simulink model "TFlex_SSGP"  (R2018b)
settings: Solver=VariableStepAuto  StartTime=0.0  StopTime=t_end  RelTol=1e-3
values from neighbouring files (symbols this model uses):
  alpha = 1    [TFlex_SSGP_init.m]
  b_init = b    [TFlex_SSGP_init.m]
  beta_init = 0.2    [TFlex_SSGP_init.m]
  beta_min = 0.0000    (= 0)    [TFlex_SSGP_init.m]
  beta_reduc = 0.9    [TFlex_SSGP_init.m]
  bufferResamp = 50    [TFlex_SSGP_init.m]
  bufferSize = 25    [TFlex_SSGP_init.m]
  hyp = abs(hyp_sn(1:end-1))    [TFlex_SSGP_init.m]
  jitter = 1e-4    (= 0.0001)    [TFlex_SSGP_init.m]
  Ma = length(b)    [TFlex_SSGP_init.m]
  ma_init = ma    [TFlex_SSGP_init.m]
  Mb = length(b)    [TFlex_SSGP_init.m]
  mu_X = mean(xTrain')    [TFlex_SSGP_init.m]
  mu_Y = mean(yTrain')    [TFlex_SSGP_init.m]
  Saa_init = Saa    [TFlex_SSGP_init.m]
  sig_X = std(xTrain')    [TFlex_SSGP_init.m]
  sig_Y = std(yTrain')    [TFlex_SSGP_init.m]
  sn = abs(hyp_sn(end))    [TFlex_SSGP_init.m]
  t_hypUpdate = [10 100]    [TFlex_SSGP_init.m]
  t_predict = 20    [TFlex_SSGP_init.m]
  ts = 1/1000    (= 0.001)    [TFlex_SSGP_init.m]
  ts_opti = ts*1000    (= 1)    [TFlex_SSGP_init.m]
  X = xTrain    [TFlex_SSGP_init.m]
  Y = yTrain    [TFlex_SSGP_init.m]
  Z = bufferSize*bufferResamp    (= 1250)    [TFlex_SSGP_init.m]
undefined symbols (not defined in the file or in its folder): Cogging, DiscIntNeverNeededParam, dof, I_limit, PID, Plant, Reference, SVF
libraries: dspmtrx3 x8, simulink x3, dspindex x2
settings Model: Creator=wout7  LastModifiedBy=wout7

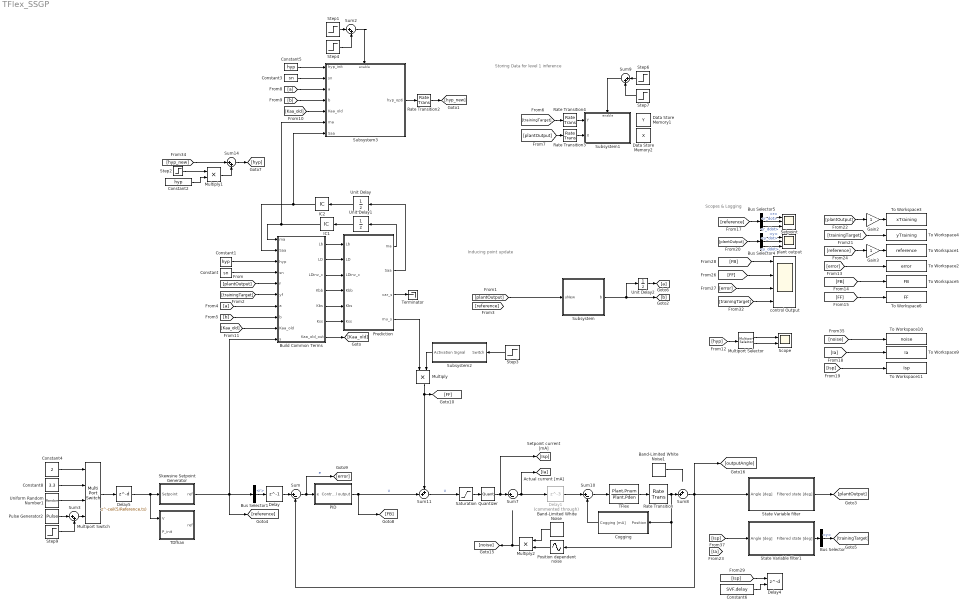
== system TFlex_SSGP ==
  note: Scopes & Logging
  note: Inducing point update
  note: Storing Data for level 1 inference
  Band-Limited White Noise : simulink/Sources/Band-Limited White Noise  Cov=[1e-3]  Ts=ts  seed=48124
  Band-Limited White Noise1 : simulink/Sources/Band-Limited White Noise  Cov=[1e-15]  Ts=ts  seed=[23341]
  Build Common Terms : Subsystem
  Bus Selector : BusSelector  OutputSignals=y
  Bus Selector1 : BusSelector  OutputSignals=r
  Bus Selector4 : BusSelector  OutputSignals=y,y_dot,y_ddot
  Bus Selector5 : BusSelector  OutputSignals=r,r_dot,r_ddot
  Cogging : Subsystem
  Constant : Constant  Value=sn
  Constant1 : Constant  Value=hyp
  Constant2 : Constant  Value=hyp  SampleTime=ts_opti
  Constant3 : Constant  Value=sn  SampleTime=ts_opti
  Constant4 : Constant  Value=2  SampleTime=Reference.ts
  Constant5 : Constant  Value=hyp
  Constant6 : Constant  Value=SVF.delay  SampleTime=ts
  Constant8 : Constant  Value=3.3  SampleTime=Reference.ts
  Data Store Memory1 : DataStoreMemory  DataStoreName=Y  ReadBeforeWriteMsg=warning  WriteAfterWriteMsg=warning  WriteAfterReadMsg=warning  InitialValue=zeros(bufferSize,1)  VectorParams1D=off  ShowAdditionalParam=off  OutDataTypeStr=double
      settings: LockScale=on
  Data Store Memory2 : DataStoreMemory  DataStoreName=X  ReadBeforeWriteMsg=warning  WriteAfterWriteMsg=warning  WriteAfterReadMsg=warning  InitialValue=zeros(bufferSize,3)  VectorParams1D=off  ShowAdditionalParam=off  OutDataTypeStr=double
      settings: LockScale=on
  Delay : Delay  DelayLength=1
  Delay1 : Delay  Commented=through  DelayLength=3  InitialCondition=0
  Delay4 : Delay  DelayLengthSource=Input port  DelayLength=3  InitialCondition=0
      settings: InputPortMap=u0,p1
  Delay5 : Delay  DelayLength=ceil(5/Reference.ts)  SampleTime=Reference.ts
  Gain2 : Gain
  Gain3 : Gain
  IC1 : InitialCondition  Value=ma_init
  IC2 : InitialCondition  Value=Saa_init
  Multiply : Product
  Multiply1 : Product
  Multiply2 : Product
  Multiport Selector : dspindex/Multiport Selector  rowsOrCols=Columns  idxCellArray={ 1:3,4}  idxErrMode=Clip Index
  Multiport Switch : MultiPortSwitch
  PID : Subsystem
  Position dependent noise : Sin  TimeSource=Use external signal  Amplitude=2.5  Bias=7.4979  Frequency=2*pi/13  SampleTime=0
  Prediction : Subsystem
  Pulse Generator2 : DiscretePulseGenerator  Amplitude=2*24  SampleTime=Reference.ts
  Quantizer : Quantizer  QuantizationInterval=1
  Rate Transition : RateTransition  OutPortSampleTime=ts
  Rate Transition2 : RateTransition  OutPortSampleTime=ts
  Rate Transition3 : RateTransition  OutPortSampleTime=ts*bufferResamp
  Rate Transition4 : RateTransition  OutPortSampleTime=ts*bufferResamp
  Saturation : Saturate  UpperLimit=I_limit  LowerLimit=-I_limit
  Scope : Scope  NumInputPorts=2
  Setpoint : Scope  NumInputPorts=3
  Skewsine Setpoint Generator : Subsystem
  State Variable filter : Subsystem
  State Variable filter1 : Subsystem
  Step1 : Step  Time=t_hypUpdate(2)  After=-1  SampleTime=ts_opti
  Step2 : Step  Time=t_hypUpdate(1)+ts  Before=1  After=0  SampleTime=ts_opti
  Step3 : Step  Time=t_predict  SampleTime=0
  Step4 : Step  Time=t_hypUpdate(1)  SampleTime=ts_opti
  Step6 : Step  Time=t_hypUpdate(2)  After=-1  SampleTime=ts_opti
  Step7 : Step  Time=t_hypUpdate(1)-Z*ts  SampleTime=ts_opti
  Step9 : Step  Time=0  After=-24  SampleTime=Reference.ts
  Subsystem : Subsystem
  Subsystem1 : Subsystem
  Subsystem2 : Subsystem
  Subsystem3 : Subsystem
  Sum : Sum  Inputs=|+-
  Sum10 : Sum  Inputs=|+-
  Sum11 : Sum  Inputs=++|
  Sum{2..3,9,14} (4 alike) : Sum  Inputs=|++
  Sum7 : Sum  Inputs=|+-
  Sum8 : Sum  Inputs=++|
  TDfhan : Subsystem
  TFlex : TransferFcn  Numerator=Plant.Pnum  Denominator=Plant.Pden  ContinuousStateAttributes='angle'
  Terminator : Terminator
  To Workspace1 : ToWorkspace  VariableName=reference  SampleTime=-1
  To Workspace10 : ToWorkspace  VariableName=noise  SampleTime=-1
  To Workspace11 : ToWorkspace  VariableName=Isp  SampleTime=-1
  To Workspace2 : ToWorkspace  VariableName=error  SampleTime=-1
  To Workspace3 : ToWorkspace  VariableName=xTraining  SampleTime=-1
  To Workspace4 : ToWorkspace  VariableName=yTraining  SampleTime=-1
  To Workspace5 : ToWorkspace  VariableName=FB  SampleTime=-1
  To Workspace6 : ToWorkspace  VariableName=FF  SampleTime=-1
  To Workspace9 : ToWorkspace  VariableName=Ia  SampleTime=-1
  Uniform Random Number1 : UniformRandomNumber  Minimum=-23  Maximum=23  Seed=Reference.seed  SampleTime=Reference.ts
  Unit Delay : UnitDelay  SampleTime=-1
  Unit Delay1 : UnitDelay  SampleTime=-1
  Unit Delay2 : UnitDelay  SampleTime=-1
  control Output : Scope  NumInputPorts=4
  plant output : Scope  NumInputPorts=3
  wires:
  Sum/1 -> [error], PID/1(e)  "e"
  Sum8/1 -> [outputAngle], Sum/2, State Variable filter/1(Angle [deg])
  Bus Selector1/1 -> Delay/1  "<r>"
  TFlex/1 -> Rate Transition/1
  [reference] -> Gain3/1
  Bus Selector5/2 -> Setpoint/2  "<r_dot>"
  Bus Selector5/1 -> Setpoint/1  "<r>"
  [error] -> To Workspace2/1
  Bus Selector5/3 -> Setpoint/3  "<r_ddot>"
  [FB] -> To Workspace5/1
  [plantOutput] -> Gain2/1
  Gain2/1 -> To Workspace3/1
  [plantOutput] -> Bus Selector4/1
  Gain3/1 -> To Workspace1/1
  Bus Selector4/1 -> plant output/1  "<y>"
  Bus Selector4/3 -> plant output/3  "<y_ddot>"
  [reference] -> Bus Selector5/1
  [trainingTarget] -> To Workspace4/1
  Bus Selector4/2 -> plant output/2  "<y_dot>"
  [FF] -> To Workspace6/1
  [trainingTarget] -> control Output/4
  [FF] -> control Output/2
  [error] -> control Output/3
  [FB] -> control Output/1
  Saturation/1 -> Quantizer/1
  PID/1(Control output) -> Sum11/2, [FB]  "u"
  State Variable filter/1(Filtered state [deg]) -> [plantOutput]
  Rate Transition/1 -> Sum8/2, Cogging/1(Position), Position dependent noise/1
  Constant6/1 -> Delay4/2
  Sum11/1 -> Saturation/1  "u"
  [Isp] -> Delay4/1
  Sum10/1 -> TFlex/1
  State Variable filter1/1(Filtered state [deg]) -> Bus Selector/1
  Sum7/1 -> Delay1/1, [Ia]
  Multiply2/1 -> [noise]
  Cogging/1(Cogging [mA]) -> Sum10/2
  Quantizer/1 -> [Isp], Sum7/1
  Multiply/1 -> Sum11/1, [FF]
  Band-Limited White Noise/1 -> Multiply2/1
  Position dependent noise/1 -> Multiply2/2
  [noise] -> To Workspace10/1
  [Ia] -> To Workspace9/1
  [Isp] -> To Workspace11/1
  Band-Limited White Noise1/1 -> ?
  Delay1/1 -> Sum10/1
  [Isp] -> State Variable filter1/1(Angle [deg])
  Prediction/1(ma) -> Unit Delay1/1
  Prediction/2(Saa) -> Unit Delay/1
  Unit Delay/1 -> IC2/1
  Unit Delay1/1 -> IC1/1
  Prediction/3(var_s) -> Terminator/1
  [plantOutput] -> Build Common Terms/5(f)
  [trainingTarget] -> Build Common Terms/6(yf)
  Constant/1 -> Build Common Terms/4(sn)
  Constant1/1 -> Build Common Terms/3(hyp)
  [a] -> Build Common Terms/7(a)
  [b] -> Build Common Terms/8(b)
  Build Common Terms/1(Lb) -> Prediction/1(Lb)
  Build Common Terms/2(LD) -> Prediction/2(LD)
  Build Common Terms/3(LDinv_c) -> Prediction/3(LDinv_c)
  Build Common Terms/4("Kbb ") -> Prediction/4(Kbb)
  Build Common Terms/5(Kbs) -> Prediction/5(Kbs)
  Build Common Terms/6(Kss) -> Prediction/6(Kss)
  Bus Selector/1 -> [trainingTarget]  "<y>"
  Unit Delay2/1 -> [a]
  IC1/1 -> Subsystem3/6(ma), Build Common Terms/1(ma)
  Prediction/4(mu_s) -> Multiply/1
  Subsystem2/1(Activation Signal) -> Multiply/2
  Step3/1 -> Subsystem2/1(Switch)
  Subsystem/1(b) -> Unit Delay2/1, [b]
  Constant8/1 -> Multiport Switch/2
  Pulse Generator2/1 -> Sum3/1
  Uniform Random Number1/1 -> Multiport Switch/3
  Sum3/1 -> Multiport Switch/4
  Multiport Switch/1 -> Delay5/1
  Step9/1 -> Sum3/2
  Constant4/1 -> Multiport Switch/1
  Delay5/1 -> Skewsine Setpoint Generator/1(Setpoint), TDfhan/1(V)
  Step7/1 -> Sum9/2
  Sum9/1 -> Subsystem1/Enable
  Rate Transition3/1 -> Subsystem1/2(X)
  Step6/1 -> Sum9/1
  [trainingTarget] -> Rate Transition4/1
  [plantOutput] -> Rate Transition3/1
  Rate Transition4/1 -> Subsystem1/1(Y)
  [a] -> Subsystem3/3(a)
  [b] -> Subsystem3/4(b)
  Build Common Terms/7(Kaa_old_out) -> [Kaa_old]
  [Kaa_old] -> Subsystem3/5(Kaa_old)
  [Kaa_old] -> Build Common Terms/9(Kaa_old)
  Subsystem3/1(hyp_opti) -> Rate Transition2/1
  Constant2/1 -> Multiply1/2
  Sum14/1 -> [hyp]
  Multiply1/1 -> Sum14/2
  [hyp_new] -> Sum14/1
  Step2/1 -> Multiply1/1
  Constant5/1 -> Subsystem3/1(hyp_init)
  Constant3/1 -> Subsystem3/2(sn)
  IC2/1 -> Subsystem3/7(Saa), Build Common Terms/2(Saa)
  Sum2/1 -> Subsystem3/Enable
  Step4/1 -> Sum2/2
  Step1/1 -> Sum2/1
  Rate Transition2/1 -> [hyp_new]
  [hyp] -> Multiport Selector/1
  Multiport Selector/1 -> Scope/1
  Multiport Selector/2 -> Scope/2
  [plantOutput] -> Subsystem/1(uNew)
  Delay/1 -> Sum/1
  Skewsine Setpoint Generator/1(ref) -> Bus Selector1/1, Build Common Terms/10(s), [reference]

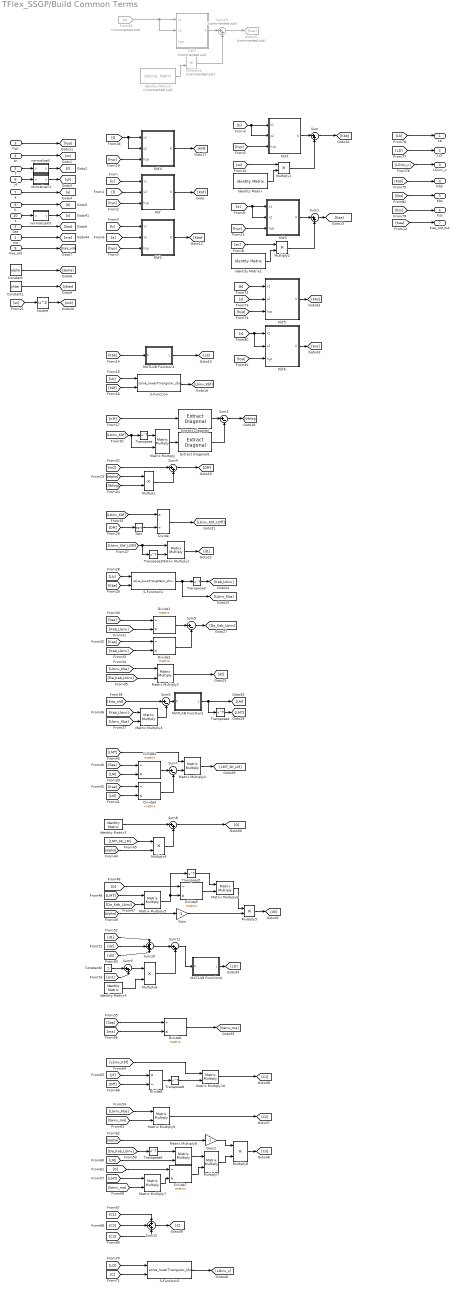
== system TFlex_SSGP/Build Common Terms ==
  ma : Inport  PortDimensions=[Ma,1]
  Saa : Inport  Port=2
  hyp : Inport  Port=3
  sn : Inport  Port=4
  f : Inport  Port=5  PortDimensions=[1,dof]
  yf : Inport  Port=6  PortDimensions=[1,1]
  a : Inport  Port=7
  b : Inport  Port=8
  Kaa_old : Inport  Port=9
  s : Inport  Port=10  PortDimensions=[1,dof]
  Constant : Constant  Value=alpha
  Constant1 : Constant  Value=jitter
  Constant2 : Constant
  Divide : Product  Inputs=*/
  Divide{1..7} (7 alike) : Product  Inputs=/*  Multiplication=Matrix(*)
  Divide8 : Product  Inputs=*/
  Extract Diagonal : dspmtrx3/Extract Diagonal
      settings: SourceProductName=DSP System Toolbox  SourceProductBaseCode=DS
  Extract Diagonal1 : dspmtrx3/Extract Diagonal
      settings: SourceProductName=DSP System Toolbox  SourceProductBaseCode=DS
  From83 : From  Commented=on  GotoTag=a
  Gain : Gain  Gain=-1
  Gain1 : Gain  Gain=-1
  Goto45 : Goto  Commented=on  GotoTag=Kaa
  Identity Matrix : dspmtrx3/Identity Matrix  Inherit=off  N=Mb  Ts=1  dataType=double  isSigned=on  wordLen=16  udDataType=sfix(16)  fracBitsMode=Best precision  numFracBits=15  OutDataTypeStr=double  LastOutDataTypeStr=double
      settings: SourceProductName=DSP System Toolbox
  Identity Matrix1 : dspmtrx3/Identity Matrix  Inherit=off  N=Ma  Ts=1  dataType=double  isSigned=on  wordLen=16  udDataType=sfix(16)  fracBitsMode=Best precision  numFracBits=15  OutDataTypeStr=double  LastOutDataTypeStr=double
      settings: SourceProductName=DSP System Toolbox
  Identity Matrix3 : dspmtrx3/Identity Matrix  Inherit=off  N=Ma  Ts=1  dataType=double  isSigned=on  wordLen=16  udDataType=sfix(16)  fracBitsMode=Best precision  numFracBits=15  OutDataTypeStr=double  LastOutDataTypeStr=double
      settings: SourceProductName=DSP System Toolbox
  Identity Matrix4 : dspmtrx3/Identity Matrix  Inherit=off  N=Mb  Ts=1  dataType=double  isSigned=on  wordLen=16  udDataType=sfix(16)  fracBitsMode=Best precision  numFracBits=15  OutDataTypeStr=double  LastOutDataTypeStr=double
      settings: SourceProductName=DSP System Toolbox
  Identity Matrix5 : dspmtrx3/Identity Matrix  Commented=on  Inherit=off  N=Mb  Ts=1  dataType=double  isSigned=on  wordLen=16  udDataType=sfix(16)  fracBitsMode=Best precision  numFracBits=15  OutDataTypeStr=double  LastOutDataTypeStr=double
      settings: SourceProductName=DSP System Toolbox
  Kbf : MATLAB Function  TreatAsAtomicUnit=on
  Kbf1 : MATLAB Function  TreatAsAtomicUnit=on
  Kbf2 : MATLAB Function  TreatAsAtomicUnit=on
  Kbf3 : MATLAB Function  TreatAsAtomicUnit=on
  Kbf4 : MATLAB Function  TreatAsAtomicUnit=on
  Kbf5 : MATLAB Function  TreatAsAtomicUnit=on
  Kbf6 : MATLAB Function  TreatAsAtomicUnit=on
  Kbf7 : MATLAB Function  Commented=on  TreatAsAtomicUnit=on
  MATLAB Function1 : MATLAB Function  TreatAsAtomicUnit=on
  MATLAB Function2 : MATLAB Function  TreatAsAtomicUnit=on
  MATLAB Function4 : MATLAB Function  TreatAsAtomicUnit=on
  Matrix Multiply{,1..10} (11 alike) : Product  Multiplication=Matrix(*)
  Multiply{,1..2,4..6,8} (7 alike) : Product
  Multiply7 : Product  Multiplication=Matrix(*)
  Multiply9 : Product  Commented=on
  S-Function : S-Function  FunctionName=solve_lowerTriangular_sfun  Parameters=Mb  SFunctionDeploymentMode=off  EnableBusSupport=off
  S-Function1 : S-Function  FunctionName=solve_lowerTriangMatrix_sfun  Parameters=Mb  SFunctionDeploymentMode=off  EnableBusSupport=off
  S-Function2 : S-Function  FunctionName=solve_lowerTriangular_sfun  Parameters=Mb  SFunctionDeploymentMode=off  EnableBusSupport=off
  Sqrt : Sqrt  SaturateOnIntegerOverflow=on
  Square : Math  Operator=square  SaturateOnIntegerOverflow=on
  Sum{,1,4,8..9,11} (6 alike) : Sum  Inputs=|++
  Sum10 : Sum  Inputs=+++
  Sum12 : Sum  Inputs=+++
  Sum13 : Sum  Commented=on  Inputs=|++
  Sum{3,5..7} (4 alike) : Sum  Inputs=|+-
  Transpose{,2..6,8} (7 alike) : Math  Operator=transpose  SaturateOnIntegerOverflow=on
  normalizeX : MATLAB Function  TreatAsAtomicUnit=on
  normalizeX3 : MATLAB Function  TreatAsAtomicUnit=on
  normalizeY1 : MATLAB Function  TreatAsAtomicUnit=on
  Lb : Outport
  LD : Outport  Port=2
  LDinv_c : Outport  Port=3
  "Kbb " : Outport  Port=4
  Kbs : Outport  Port=5
  Kss : Outport  Port=6
  Kaa_old_out : Outport  Port=7
  wires:
  Saa/1 -> [Saa]
  yf/1 -> normalizeY1/1(u)
  f/1 -> normalizeX/1(u)
  sn/1 -> [sn]
  hyp/1 -> [hyp]
  Constant/1 -> [alpha]
  Constant1/1 -> [jitter]
  [b] -> Kbf/1(x1)
  [f] -> Kbf/2(x2)
  [hyp] -> Kbf/3(hyp)
  Kbf/1(K) -> [Kbf]
  [hyp] -> Kbf1/3(hyp)
  [b] -> Kbf1/2(x2), Kbf1/1(x1)
  Multiply1/1 -> Sum/2
  Identity Matrix/1 -> Multiply1/2
  [sn] -> Multiply1/1
  Kbf1/1(K) -> Sum/1
  Sum/1 -> [Kbb]
  [hyp] -> Kbf2/3(hyp)
  [a] -> Kbf2/2(x2)
  [b] -> Kbf2/1(x1)
  Kbf2/1(K) -> [Kba]
  [hyp] -> Kbf3/3(hyp)
  [a] -> Kbf3/2(x2), Kbf3/1(x1)
  Multiply2/1 -> Sum1/2
  [sn] -> Multiply2/1
  Identity Matrix1/1 -> Multiply2/2
  Kbf3/1(K) -> Sum1/1
  Sum1/1 -> [Kaa]
  [Kbb] -> MATLAB Function1/1(K)
  MATLAB Function1/1(L) -> [Lb]
  [Lb] -> S-Function/1
  [Kbf] -> S-Function/2
  S-Function/1 -> [Lbinv_Kbf]
  [hyp] -> Kbf4/3(hyp)
  Kbf4/1(K) -> [Kff]
  [f] -> Kbf4/2(x2), Kbf4/1(x1)
  [Kff] -> Extract Diagonal/1
  [Lbinv_Kbf] -> Matrix Multiply/2, Transpose/1
  Transpose/1 -> Matrix Multiply/1
  Matrix Multiply/1 -> Extract Diagonal1/1
  Extract Diagonal/1 -> Sum3/1
  Sum3/1 -> [Qfdiag]
  Extract Diagonal1/1 -> Sum3/2
  [sn] -> Square/1
  Square/1 -> [sn2]
  [alpha] -> Multiply/1
  [Qfdiag] -> Multiply/2
  Multiply/1 -> Sum4/2
  [sn2] -> Sum4/1
  Sum4/1 -> [Dff]
  [Lbinv_Kbf] -> Divide/1
  Sqrt/1 -> Divide/2
  Divide/1 -> [Lbinv_Kbf_LDff]
  Transpose2/1 -> Matrix Multiply1/2
  [Lbinv_Kbf_LDff] -> Transpose2/1, Matrix Multiply1/1
  Matrix Multiply1/1 -> [d1]
  [Lb] -> S-Function1/1
  [Kba] -> S-Function1/2
  Transpose3/1 -> [Kab_Lbinv]
  S-Function1/1 -> Transpose3/1, [Lbinv_Kba]
  [Saa] -> Divide1/1
  [Kab_Lbinv] -> Divide1/2
  Divide1/1 -> Sum5/1
  Divide2/1 -> Sum5/2
  [Kab_Lbinv] -> Divide2/2
  [Kaa] -> Divide2/1
  Sum5/1 -> [Da_Kab_Lbinv]
  [Da_Kab_Lbinv] -> Matrix Multiply2/2
  [Lbinv_Kba] -> Matrix Multiply2/1
  Matrix Multiply2/1 -> [d2]
  [Lbinv_Kba] -> Matrix Multiply3/2
  [Kab_Lbinv] -> Matrix Multiply3/1
  Matrix Multiply3/1 -> Sum6/2
  [Kaa_old] -> Sum6/1
  Sum6/1 -> MATLAB Function2/1(K)
  MATLAB Function2/1(L) -> [LM], Transpose4/1
  Transpose4/1 -> [LMT]
  [LM] -> Divide3/2
  [Saa] -> Divide3/1
  [Kaa] -> Divide4/1
  [LM] -> Divide4/2
  Divide3/1 -> Sum7/1
  Divide4/1 -> Sum7/2
  Sum7/1 -> Matrix Multiply4/2
  Matrix Multiply4/1 -> [LMT_SK_LM]
  [LMT] -> Matrix Multiply4/1
  Identity Matrix3/1 -> Sum8/1
  [alpha] -> Multiply4/2
  [LMT_SK_LM] -> Multiply4/1
  Multiply4/1 -> Sum8/2
  Sum8/1 -> [Q]
  [LMT] -> Matrix Multiply5/1
  [Da_Kab_Lbinv] -> Matrix Multiply5/2
  Matrix Multiply5/1 -> Transpose5/1, Divide5/2
  [Q] -> Divide5/1
  Divide5/1 -> Matrix Multiply6/2
  Transpose5/1 -> Matrix Multiply6/1
  Matrix Multiply6/1 -> Multiply5/1
  [alpha] -> Gain/1
  Gain/1 -> Multiply5/2
  Multiply5/1 -> [d3]
  Constant2/1 -> Sum9/1
  [sn2] -> Sum9/2
  Sum9/1 -> Multiply6/1
  Identity Matrix4/1 -> Multiply6/2
  [d2] -> Sum10/2
  [d3] -> Sum10/3
  [d1] -> Sum10/1
  Sum10/1 -> Sum11/1
  Multiply6/1 -> Sum11/2
  Sum11/1 -> MATLAB Function4/1(K)
  MATLAB Function4/1(L) -> [LD]
  [Saa] -> Divide6/1
  [ma] -> Divide6/2
  Divide6/1 -> [Sainv_ma]
  [LMT] -> Matrix Multiply7/1
  [Sainv_ma] -> Matrix Multiply7/2
  [Da_Kab_Lbinv] -> Transpose6/1
  Transpose6/1 -> Matrix Multiply8/1
  [LM] -> Matrix Multiply8/2
  [Q] -> Divide7/1
  Matrix Multiply7/1 -> Divide7/2
  Matrix Multiply8/1 -> Multiply7/1
  Divide7/1 -> Multiply7/2
  Multiply7/1 -> Multiply8/2
  [alpha] -> Gain1/1
  Gain1/1 -> Multiply8/1
  Multiply8/1 -> [C3]
  [Lbinv_Kba] -> Matrix Multiply9/1
  [Sainv_ma] -> Matrix Multiply9/2
  Matrix Multiply9/1 -> [C2]
  [yf] -> Divide8/1
  [Dff] -> Divide8/2
  Divide8/1 -> Transpose8/1
  [Lbinv_Kbf] -> Matrix Multiply10/1
  Transpose8/1 -> Matrix Multiply10/2
  Matrix Multiply10/1 -> [C1]
  [C2] -> Sum12/2
  [C1] -> Sum12/1
  [C3] -> Sum12/3
  Sum12/1 -> [C]
  [LD] -> S-Function2/1
  [C] -> S-Function2/2
  S-Function2/1 -> [LDinv_c]
  s/1 -> normalizeX3/1(u)
  [b] -> Kbf5/1(x1)
  [s] -> Kbf5/2(x2)
  [hyp] -> Kbf5/3(hyp)
  Kbf5/1(K) -> [Kbs]
  [Kbb] -> "Kbb "/1
  [LDinv_c] -> LDinv_c/1
  [LD] -> LD/1
  [Lb] -> Lb/1
  [Kbs] -> Kbs/1
  a/1 -> [a]
  b/1 -> [b]
  normalizeX3/1(y) -> [s]
  ma/1 -> [ma]
  normalizeY1/1(y) -> [yf]
  [Dff] -> Sqrt/1
  Kbf6/1(K) -> [Kss]
  [hyp] -> Kbf6/3(hyp)
  [s] -> Kbf6/1(x1), Kbf6/2(x2)
  [Kss] -> Kss/1
  ? -> Kbf7/3(hyp)
  Identity Matrix5/1 -> Multiply9/2
  From83/1 -> Kbf7/2(x2), Kbf7/1(x1)
  Multiply9/1 -> Sum13/2
  ? -> Multiply9/1
  Kbf7/1(K) -> Sum13/1
  Sum13/1 -> Goto45/1
  normalizeX/1(y) -> [f]
  Kaa_old/1 -> [Kaa_old]
  [Kaa] -> Kaa_old_out/1

== system TFlex_SSGP/Cogging ==
  Position : Inport
  Gain : Gain  Gain=20
  Scope : Scope
  Sine Wave Function : Sin  TimeSource=Use external signal  Amplitude=Cogging.amplitude  Frequency=2*pi./Cogging.frequency  Phase=Cogging.phase*2*pi  SampleTime=0
  Sum of Elements : Sum  Inputs=+
  Cogging [mA] : Outport
  wires:
  Gain/1 -> Scope/1, [Cogging], Cogging [mA]/1
  Sum of Elements/1 -> Gain/1
  Position/1 -> Sine Wave Function/1
  Sine Wave Function/1 -> Sum of Elements/1

== system TFlex_SSGP/PID ==
  e : Inport
  Discrete Derivative : simulink/Discrete/Discrete Derivative  gainval=1.0  ICPrevScaledInput=0.0  OutMin=[]  OutMax=[]  OutDataType=fixdt(1, 16)  OutScaling=2^-10  DoSatur=off
  Discrete-Time Integrator2 : DiscreteIntegrator  SampleTime=-1  ICPrevOutput=DiscIntNeverNeededParam  ICPrevScaledInput=DiscIntNeverNeededParam
  Gain1 : Gain  Gain=PID.Kp
  Gain2 : Gain  Gain=PID.Ki
  Gain3 : Gain  Gain=PID.Kd
  Lowpass : DiscreteTransferFcn  Numerator=PID.LPnum  Denominator=PID.LPden  SampleTime=ts
  Sum2 : Sum  Inputs=3
  Control output : Outport
  wires:
  Discrete-Time Integrator2/1 -> Gain2/1
  Gain1/1 -> Sum2/2
  Gain2/1 -> Sum2/1
  Gain3/1 -> Sum2/3
  Sum2/1 -> Control output/1
  e/1 -> Discrete-Time Integrator2/1, Gain1/1, Lowpass/1
  Lowpass/1 -> Discrete Derivative/1
  Discrete Derivative/1 -> Gain3/1

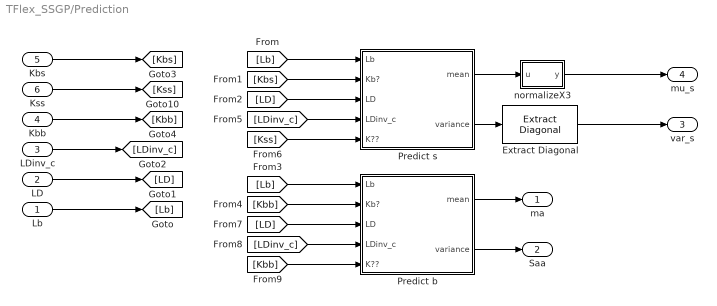
== system TFlex_SSGP/Prediction ==
  Lb : Inport
  LD : Inport  Port=2
  LDinv_c : Inport  Port=3
  Kbb : Inport  Port=4
  Kbs : Inport  Port=5
  Kss : Inport  Port=6
  Extract Diagonal : dspmtrx3/Extract Diagonal
      settings: SourceProductName=DSP System Toolbox  SourceProductBaseCode=DS
  Predict b : Subsystem
  Predict s : Subsystem
  normalizeX3 : MATLAB Function  TreatAsAtomicUnit=on
  ma : Outport
  Saa : Outport  Port=2
  var_s : Outport  Port=3
  mu_s : Outport  Port=4
  wires:
  Kbs/1 -> [Kbs]
  Kss/1 -> [Kss]
  Extract Diagonal/1 -> var_s/1
  [Lb] -> Predict s/1(Lb)
  [Kbs] -> Predict s/2(Kb?)
  [LD] -> Predict s/3(LD)
  [LDinv_c] -> Predict s/4(LDinv_c)
  [Kss] -> Predict s/5(K??)
  Predict s/1(mean) -> normalizeX3/1(u)
  Predict s/2(variance) -> Extract Diagonal/1
  [Kbb] -> Predict b/2(Kb?)
  [Kbb] -> Predict b/5(K??)
  [LDinv_c] -> Predict b/4(LDinv_c)
  [LD] -> Predict b/3(LD)
  Predict b/2(variance) -> Saa/1
  [Lb] -> Predict b/1(Lb)
  Predict b/1(mean) -> ma/1
  Lb/1 -> [Lb]
  Kbb/1 -> [Kbb]
  LDinv_c/1 -> [LDinv_c]
  LD/1 -> [LD]
  normalizeX3/1(y) -> mu_s/1

== system TFlex_SSGP/Skewsine Setpoint Generator ==
  Setpoint : Inport
  Bus Creator : BusCreator  Inputs=3
  Subsystem : Subsystem
  ref : Outport
  wires:
  Subsystem/3(r_ddot) -> Bus Creator/3  "r_ddot"
  Bus Creator/1 -> ref/1
  Subsystem/2(r_dot) -> Bus Creator/2  "r_dot"
  Subsystem/1(r) -> Bus Creator/1  "r"
  Setpoint/1 -> Subsystem/1(setpoint)

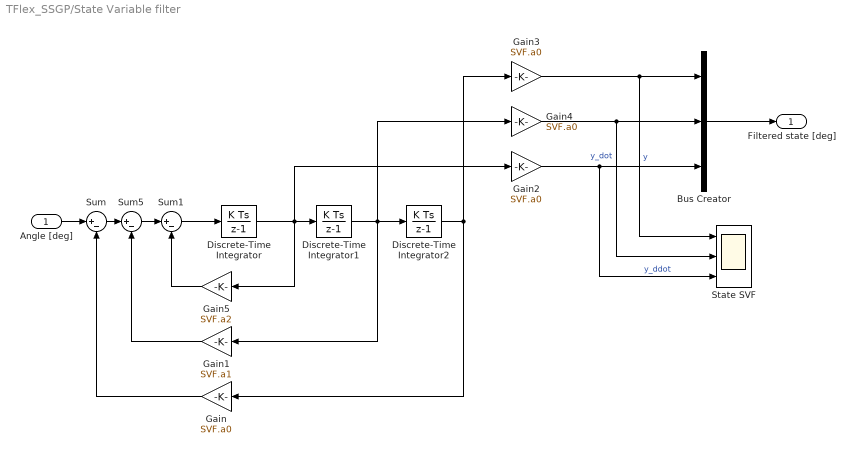
== system TFlex_SSGP/State Variable filter ==
  Angle [deg] : Inport
  Bus Creator : BusCreator  Inputs=3
  Discrete-Time Integrator : DiscreteIntegrator  SampleTime=-1  ICPrevOutput=DiscIntNeverNeededParam  ICPrevScaledInput=DiscIntNeverNeededParam
  Discrete-Time Integrator1 : DiscreteIntegrator  SampleTime=-1  ICPrevOutput=DiscIntNeverNeededParam  ICPrevScaledInput=DiscIntNeverNeededParam
  Discrete-Time Integrator2 : DiscreteIntegrator  SampleTime=-1  ICPrevOutput=DiscIntNeverNeededParam  ICPrevScaledInput=DiscIntNeverNeededParam
  Gain{,2..4} (4 alike) : Gain  Gain=SVF.a0
  Gain1 : Gain  Gain=SVF.a1
  Gain5 : Gain  Gain=SVF.a2
  State SVF : Scope  NumInputPorts=3
  Sum : Sum  Inputs=|+-
  Sum1 : Sum  Inputs=|+-
  Sum5 : Sum  Inputs=|+-
  Filtered state [deg] : Outport  SampleTime=ts
  wires:
  Bus Creator/1 -> Filtered state [deg]/1
  Sum1/1 -> Discrete-Time Integrator/1
  Angle [deg]/1 -> Sum/1
  Sum/1 -> Sum5/1
  Gain/1 -> Sum/2
  Gain1/1 -> Sum5/2
  Gain3/1 -> State SVF/1, Bus Creator/1  "y"
  Gain2/1 -> State SVF/3, Bus Creator/3  "y_ddot"
  Gain4/1 -> State SVF/2, Bus Creator/2  "y_dot"
  Gain5/1 -> Sum1/2
  Sum5/1 -> Sum1/1
  Discrete-Time Integrator/1 -> Discrete-Time Integrator1/1, Gain2/1, Gain5/1
  Discrete-Time Integrator1/1 -> Discrete-Time Integrator2/1, Gain4/1, Gain1/1
  Discrete-Time Integrator2/1 -> Gain3/1, Gain/1

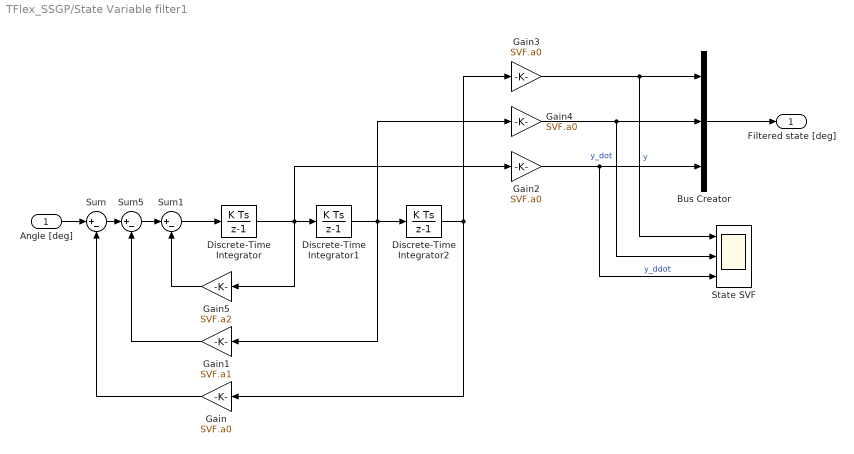
== system TFlex_SSGP/State Variable filter1 ==
  Angle [deg] : Inport
  Bus Creator : BusCreator  Inputs=3
  Discrete-Time Integrator : DiscreteIntegrator  SampleTime=-1  ICPrevOutput=DiscIntNeverNeededParam  ICPrevScaledInput=DiscIntNeverNeededParam
  Discrete-Time Integrator1 : DiscreteIntegrator  SampleTime=-1  ICPrevOutput=DiscIntNeverNeededParam  ICPrevScaledInput=DiscIntNeverNeededParam
  Discrete-Time Integrator2 : DiscreteIntegrator  SampleTime=-1  ICPrevOutput=DiscIntNeverNeededParam  ICPrevScaledInput=DiscIntNeverNeededParam
  Gain{,2..4} (4 alike) : Gain  Gain=SVF.a0
  Gain1 : Gain  Gain=SVF.a1
  Gain5 : Gain  Gain=SVF.a2
  State SVF : Scope  NumInputPorts=3
  Sum : Sum  Inputs=|+-
  Sum1 : Sum  Inputs=|+-
  Sum5 : Sum  Inputs=|+-
  Filtered state [deg] : Outport  SampleTime=ts
  wires:
  Bus Creator/1 -> Filtered state [deg]/1
  Sum1/1 -> Discrete-Time Integrator/1
  Angle [deg]/1 -> Sum/1
  Sum/1 -> Sum5/1
  Gain/1 -> Sum/2
  Gain1/1 -> Sum5/2
  Gain3/1 -> State SVF/1, Bus Creator/1  "y"
  Gain2/1 -> State SVF/3, Bus Creator/3  "y_ddot"
  Gain4/1 -> State SVF/2, Bus Creator/2  "y_dot"
  Gain5/1 -> Sum1/2
  Sum5/1 -> Sum1/1
  Discrete-Time Integrator/1 -> Discrete-Time Integrator1/1, Gain2/1, Gain5/1
  Discrete-Time Integrator1/1 -> Discrete-Time Integrator2/1, Gain4/1, Gain1/1
  Discrete-Time Integrator2/1 -> Gain3/1, Gain/1

== system TFlex_SSGP/Subsystem ==
  uNew : Inport  PortDimensions=[1,dof]
  Constant : Constant  Value=[2:Mb]
  IC1 : InitialCondition  Value=b_init
  Matrix Concatenate4 : Concatenate  Mode=Multidimensional array
  Subsystem : Subsystem
  Unit Delay : UnitDelay  SampleTime=-1
  Variable Selector5 : dspindex/Variable Selector  NumInputs=1  rowsOrCols=Rows  IdxMode=Variable  Elements=[1 3]  ZerOneIdxMode=One-based  errmode=Clip Index  FillMode=off  FillValues=0
  normalizeX1 : MATLAB Function  TreatAsAtomicUnit=on
  b : Outport
  wires:
  Variable Selector5/1 -> Matrix Concatenate4/1
  uNew/1 -> normalizeX1/1(u)
  Unit Delay/1 -> Variable Selector5/1
  Matrix Concatenate4/1 -> IC1/1
  [b] -> b/1
  IC1/1 -> Unit Delay/1, [b]
  normalizeX1/1(y) -> Matrix Concatenate4/2
  Constant/1 -> Variable Selector5/2

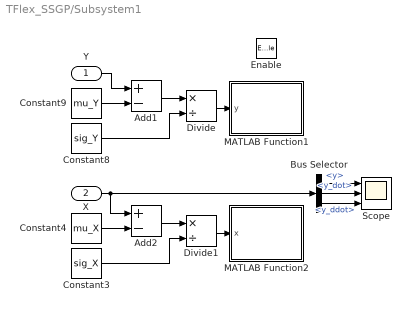
== system TFlex_SSGP/Subsystem1 ==
  Y : Inport
  X : Inport  Port=2
  Enable : EnablePort
  Add1 : Sum  Inputs=+-
  Add2 : Sum  Inputs=+-
  Bus Selector : BusSelector  OutputSignals=y,y_dot,y_ddot
  Constant3 : Constant  Value=sig_X  VectorParams1D=off  SampleTime=ts_opti
  Constant4 : Constant  Value=mu_X  VectorParams1D=off  SampleTime=ts_opti
  Constant8 : Constant  Value=sig_Y  VectorParams1D=off  SampleTime=ts_opti
  Constant9 : Constant  Value=mu_Y  VectorParams1D=off  SampleTime=ts_opti
  Divide : Product  Inputs=*/
  Divide1 : Product  Inputs=*/
  MATLAB Function1 : MATLAB Function  TreatAsAtomicUnit=on
  MATLAB Function2 : MATLAB Function  TreatAsAtomicUnit=on
  Scope : Scope  NumInputPorts=3
  wires:
  Divide1/1 -> MATLAB Function2/1(x)
  Y/1 -> Add1/1
  Divide/1 -> MATLAB Function1/1(y)
  Add1/1 -> Divide/1
  Add2/1 -> Divide1/1
  Constant9/1 -> Add1/2
  Constant3/1 -> Divide1/2
  Constant4/1 -> Add2/2
  Constant8/1 -> Divide/2
  Bus Selector/1 -> Scope/1  "<y>"
  Bus Selector/2 -> Scope/2  "<y_dot>"
  Bus Selector/3 -> Scope/3  "<y_ddot>"
  X/1 -> Add2/1, Bus Selector/1

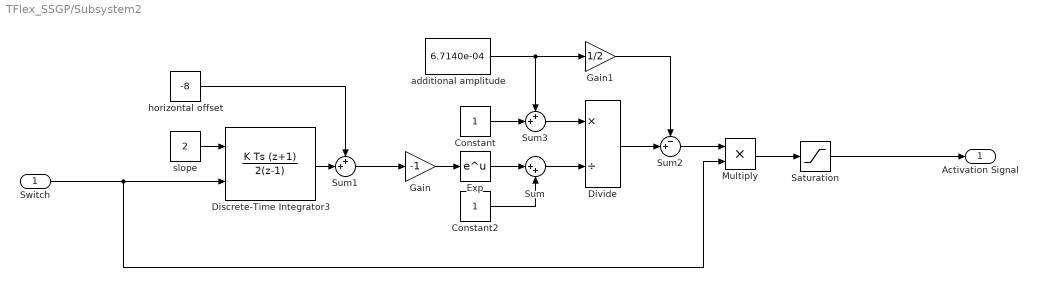
== system TFlex_SSGP/Subsystem2 ==
  Switch : Inport
  Constant : Constant
  Constant2 : Constant
  Discrete-Time Integrator3 : DiscreteIntegrator  IntegratorMethod=Integration: Trapezoidal  ExternalReset=rising  SampleTime=-1  UpperSaturationLimit=1  LowerSaturationLimit=0  ICPrevOutput=DiscIntNeverNeededParam  ICPrevScaledInput=DiscIntNeverNeededParam
  Divide : Product  Inputs=*/
  Exp : Math  SaturateOnIntegerOverflow=on
  Gain : Gain  Gain=-1
  Gain1 : Gain  Gain=1/2
  Multiply : Product
  Saturation : Saturate  UpperLimit=1  LowerLimit=0
  Sum : Sum  Inputs=|++
  Sum1 : Sum  Inputs=++|
  Sum2 : Sum  Inputs=-+|
  Sum3 : Sum  Inputs=++|
  additional amplitude : Constant  Value=6.7140e-04
  horizontal offset : Constant  Value=-8
  slope : Constant  Value=2
  Activation Signal : Outport
  wires:
  Constant/1 -> Sum3/2
  Exp/1 -> Sum/1
  additional amplitude/1 -> Sum3/1, Gain1/1
  Sum1/1 -> Gain/1
  Gain1/1 -> Sum2/1
  Divide/1 -> Sum2/2
  Sum/1 -> Divide/2
  Gain/1 -> Exp/1
  slope/1 -> Discrete-Time Integrator3/1
  Discrete-Time Integrator3/1 -> Sum1/2
  Constant2/1 -> Sum/2
  Sum2/1 -> Multiply/1
  Sum3/1 -> Divide/1
  horizontal offset/1 -> Sum1/1
  Saturation/1 -> Activation Signal/1
  Multiply/1 -> Saturation/1
  Switch/1 -> Multiply/2, Discrete-Time Integrator3/2

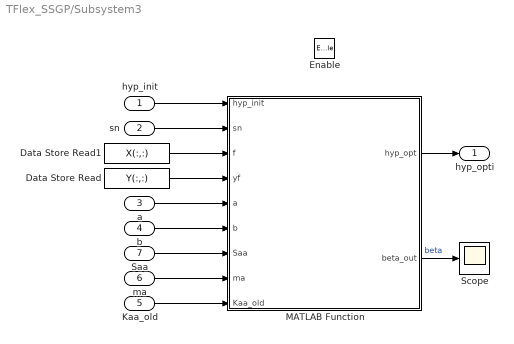
== system TFlex_SSGP/Subsystem3 ==
  hyp_init : Inport  PortDimensions=[1,4]
  sn : Inport  Port=2
  a : Inport  Port=3
  b : Inport  Port=4
  Kaa_old : Inport  Port=5
  ma : Inport  Port=6
  Saa : Inport  Port=7
  Enable : EnablePort
  Data Store Read : DataStoreRead  DataStoreName=Y  SampleTime=ts_opti  DataStoreElements=Y(:,:)
  Data Store Read1 : DataStoreRead  DataStoreName=X  SampleTime=ts_opti  DataStoreElements=X(:,:)
  MATLAB Function : MATLAB Function  TreatAsAtomicUnit=on
  Scope : Scope
  hyp_opti : Outport
  wires:
  hyp_init/1 -> MATLAB Function/1(hyp_init)
  MATLAB Function/2(beta_out) -> Scope/1  "beta"
  sn/1 -> MATLAB Function/2(sn)
  MATLAB Function/1(hyp_opt) -> hyp_opti/1
  Data Store Read/1 -> MATLAB Function/4(yf)
  Data Store Read1/1 -> MATLAB Function/3(f)
  a/1 -> MATLAB Function/5(a)
  b/1 -> MATLAB Function/6(b)
  ma/1 -> MATLAB Function/8(ma)
  Kaa_old/1 -> MATLAB Function/9(Kaa_old)
  Saa/1 -> MATLAB Function/7(Saa)

== system TFlex_SSGP/TDfhan ==
  V : Inport
  P_init : Inport  Port=2
  Bus Creator : BusCreator  Inputs=3
  Constant : Constant  Value=Reference.transient.r  SampleTime=ts
  Constant1 : Constant  Value=Reference.transient.h  SampleTime=ts
  Discrete-Time Integrator : DiscreteIntegrator  gainval=1  SampleTime=ts  ICPrevOutput=DiscIntNeverNeededParam  ICPrevScaledInput=DiscIntNeverNeededParam
  Discrete-Time Integrator1 : DiscreteIntegrator  gainval=1  InitialConditionSource=external  InitialCondition=-24  SampleTime=ts  ICPrevOutput=DiscIntNeverNeededParam  ICPrevScaledInput=DiscIntNeverNeededParam
  MATLAB Function2 : MATLAB Function  TreatAsAtomicUnit=on
  Scope : Scope  NumInputPorts=3
  Sum : Sum  Inputs=+-|
  ref : Outport
  wires:
  Sum/1 -> MATLAB Function2/1(v1)
  V/1 -> Sum/2
  Constant/1 -> MATLAB Function2/3(r0)
  Constant1/1 -> MATLAB Function2/4(h0)
  P_init/1 -> Discrete-Time Integrator1/2
  Discrete-Time Integrator1/1 -> Sum/1, Scope/1, Bus Creator/1  "r"
  Discrete-Time Integrator/1 -> Discrete-Time Integrator1/1, Scope/2, Bus Creator/2, MATLAB Function2/2(v2)  "r_dot"
  Bus Creator/1 -> ref/1
  MATLAB Function2/1(output) -> Scope/3, Bus Creator/3, Discrete-Time Integrator/1  "r_ddot"

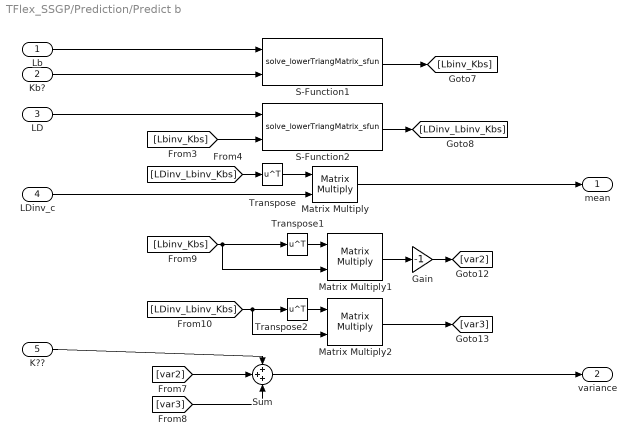
== system TFlex_SSGP/Prediction/Predict b ==
  Lb : Inport
  Kb? : Inport  Port=2
  LD : Inport  Port=3
  LDinv_c : Inport  Port=4
  K?? : Inport  Port=5
  Gain : Gain  Gain=-1
  Matrix Multiply : Product  Multiplication=Matrix(*)
  Matrix Multiply1 : Product  Multiplication=Matrix(*)
  Matrix Multiply2 : Product  Multiplication=Matrix(*)
  S-Function1 : S-Function  FunctionName=solve_lowerTriangMatrix_sfun  Parameters=Mb  SFunctionDeploymentMode=off  EnableBusSupport=off
  S-Function2 : S-Function  FunctionName=solve_lowerTriangMatrix_sfun  Parameters=Mb  SFunctionDeploymentMode=off  EnableBusSupport=off
  Sum : Sum  Inputs=+++
  Transpose : Math  Operator=transpose  SaturateOnIntegerOverflow=on
  Transpose1 : Math  Operator=transpose  SaturateOnIntegerOverflow=on
  Transpose2 : Math  Operator=transpose  SaturateOnIntegerOverflow=on
  mean : Outport
  variance : Outport  Port=2
  wires:
  Transpose2/1 -> Matrix Multiply2/1
  Lb/1 -> S-Function1/1
  S-Function2/1 -> [LDinv_Lbinv_Kbs]
  Transpose1/1 -> Matrix Multiply1/1
  Matrix Multiply2/1 -> [var3]
  [var3] -> Sum/3
  [Lbinv_Kbs] -> S-Function2/2
  Matrix Multiply1/1 -> Gain/1
  [LDinv_Lbinv_Kbs] -> Matrix Multiply2/2, Transpose2/1
  [Lbinv_Kbs] -> Matrix Multiply1/2, Transpose1/1
  S-Function1/1 -> [Lbinv_Kbs]
  [var2] -> Sum/2
  [LDinv_Lbinv_Kbs] -> Transpose/1
  LDinv_c/1 -> Matrix Multiply/2
  Matrix Multiply/1 -> mean/1
  Transpose/1 -> Matrix Multiply/1
  Sum/1 -> variance/1
  Kb?/1 -> S-Function1/2
  LD/1 -> S-Function2/1
  K??/1 -> Sum/1
  Gain/1 -> [var2]

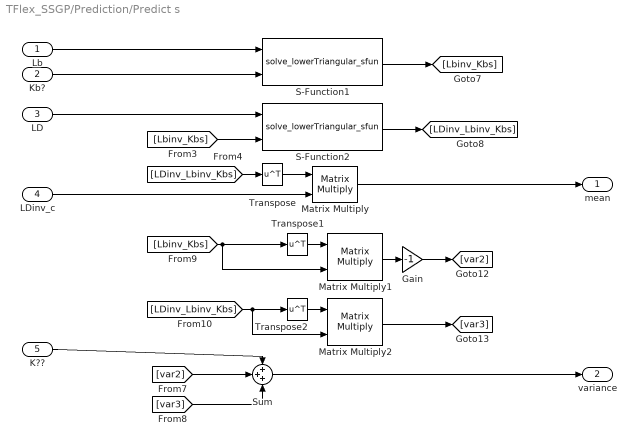
== system TFlex_SSGP/Prediction/Predict s ==
  Lb : Inport
  Kb? : Inport  Port=2
  LD : Inport  Port=3
  LDinv_c : Inport  Port=4
  K?? : Inport  Port=5
  Gain : Gain  Gain=-1
  Matrix Multiply : Product  Multiplication=Matrix(*)
  Matrix Multiply1 : Product  Multiplication=Matrix(*)
  Matrix Multiply2 : Product  Multiplication=Matrix(*)
  S-Function1 : S-Function  FunctionName=solve_lowerTriangular_sfun  Parameters=Mb  SFunctionDeploymentMode=off  EnableBusSupport=off
  S-Function2 : S-Function  FunctionName=solve_lowerTriangular_sfun  Parameters=Mb  SFunctionDeploymentMode=off  EnableBusSupport=off
  Sum : Sum  Inputs=+++
  Transpose : Math  Operator=transpose  SaturateOnIntegerOverflow=on
  Transpose1 : Math  Operator=transpose  SaturateOnIntegerOverflow=on
  Transpose2 : Math  Operator=transpose  SaturateOnIntegerOverflow=on
  mean : Outport
  variance : Outport  Port=2
  wires:
  Transpose2/1 -> Matrix Multiply2/1
  Lb/1 -> S-Function1/1
  S-Function2/1 -> [LDinv_Lbinv_Kbs]
  Transpose1/1 -> Matrix Multiply1/1
  Matrix Multiply2/1 -> [var3]
  [var3] -> Sum/3
  [Lbinv_Kbs] -> S-Function2/2
  Matrix Multiply1/1 -> Gain/1
  [LDinv_Lbinv_Kbs] -> Matrix Multiply2/2, Transpose2/1
  [Lbinv_Kbs] -> Transpose1/1, Matrix Multiply1/2
  S-Function1/1 -> [Lbinv_Kbs]
  [var2] -> Sum/2
  [LDinv_Lbinv_Kbs] -> Transpose/1
  LDinv_c/1 -> Matrix Multiply/2
  Matrix Multiply/1 -> mean/1
  Transpose/1 -> Matrix Multiply/1
  Sum/1 -> variance/1
  Kb?/1 -> S-Function1/2
  LD/1 -> S-Function2/1
  K??/1 -> Sum/1
  Gain/1 -> [var2]

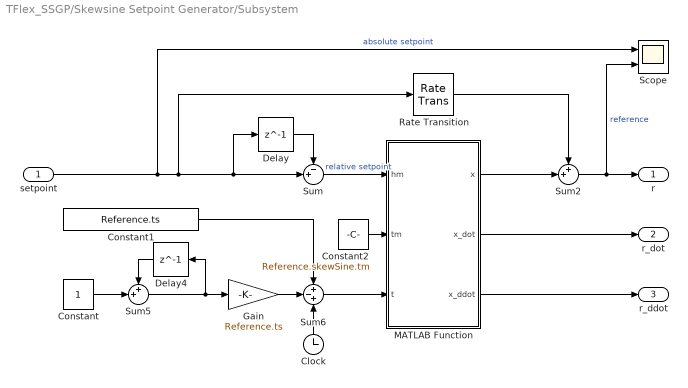
== system TFlex_SSGP/Skewsine Setpoint Generator/Subsystem ==
  setpoint : Inport
  Clock : Clock
      settings: Decimation=100
  Constant : Constant  SampleTime=Reference.ts
  Constant1 : Constant  Value=Reference.ts  SampleTime=Reference.ts
  Constant2 : Constant  Value=Reference.skewSine.tm  SampleTime=Reference.ts
  Delay : Delay  DelayLength=1  InitialCondition=0  SampleTime=Reference.ts
  Delay4 : Delay  DelayLength=1  InitialCondition=0  SampleTime=Reference.ts
  Gain : Gain  Gain=Reference.ts
  MATLAB Function : MATLAB Function  TreatAsAtomicUnit=on
  Rate Transition : RateTransition  OutPortSampleTime=ts
  Scope : Scope  NumInputPorts=2
  Sum : Sum  Inputs=-+|
  Sum2 : Sum  Inputs=++|
  Sum5 : Sum  Inputs=++|
  Sum6 : Sum  Inputs=+-+
  r : Outport
  r_dot : Outport  Port=2
  r_ddot : Outport  Port=3
  wires:
  Delay4/1 -> Sum5/1
  Sum2/1 -> r/1, Scope/2  "reference"
  Sum5/1 -> Delay4/1, Gain/1
  Constant/1 -> Sum5/2
  MATLAB Function/3(x_ddot) -> r_ddot/1
  Clock/1 -> Sum6/3
  Delay/1 -> Sum/1
  Gain/1 -> Sum6/2
  Constant1/1 -> Sum6/1
  MATLAB Function/2(x_dot) -> r_dot/1
  Sum/1 -> MATLAB Function/1(hm)  "relative setpoint"
  Constant2/1 -> MATLAB Function/2(tm)
  Sum6/1 -> MATLAB Function/3(t)
  MATLAB Function/1(x) -> Sum2/2
  setpoint/1 -> Scope/1, Rate Transition/1, Delay/1, Sum/2  "absolute setpoint"
  Rate Transition/1 -> Sum2/1

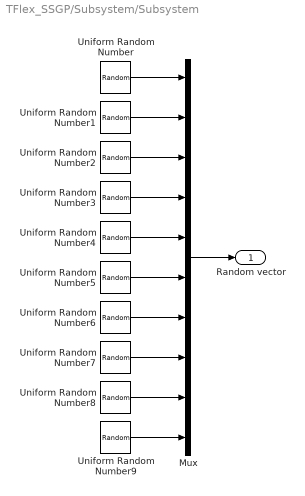
== system TFlex_SSGP/Subsystem/Subsystem ==
  Mux : Mux  Inputs=10
  Uniform Random Number{,1..9} (10 alike) : UniformRandomNumber  Minimum=1  Maximum=Mb  Seed=randi(2000,1)  SampleTime=ts
  Random vector : Outport
  wires:
  Uniform Random Number/1 -> Mux/1
  Mux/1 -> Random vector/1
  Uniform Random Number1/1 -> Mux/2
  Uniform Random Number2/1 -> Mux/3
  Uniform Random Number3/1 -> Mux/4
  Uniform Random Number4/1 -> Mux/5
  Uniform Random Number5/1 -> Mux/6
  Uniform Random Number6/1 -> Mux/7
  Uniform Random Number7/1 -> Mux/8
  Uniform Random Number8/1 -> Mux/9
  Uniform Random Number9/1 -> Mux/10

== matlab function TFlex_SSGP/Build Common Terms/Kbf7 ==
  data: x1 input; K output size=[Nkeep+1,Nkeep+1]; x2 input; hyp input
function K = SquaredExpCov(x1,x2,hyp) %#codegen
coder.extrinsic('SEcov');
n = size(x1,1);
K = double(zeros(n));
K = SEcov(x1,x2,hyp);
end

== matlab function TFlex_SSGP/Skewsine Setpoint Generator/Subsystem/MATLAB Function ==
  settings: updateMethod=DISCRETE  sampleTime=ts
  data: hm input; x output; tm input; t input; x_dot output; x_ddot output
function [x,x_dot,x_ddot] = skewSine(hm,tm,t)

if (t>=0) && (t<=tm)
    x      = hm/tm*t - hm/(2*pi)*sin(2*pi/tm*t);
    x_dot  = hm/tm - hm/tm*cos(2*pi/tm*t);
    x_ddot = 2*pi*hm/(tm^2)*sin(2*pi/tm*t);
else
    x      = hm;
    x_dot  = 0;
    x_ddot = 0;
end

== matlab function TFlex_SSGP/Build Common Terms/normalizeX ==
  data: u input; y output size=[1,dof]; mu_X parameter; sig_X parameter
function y = normalizeX(u,mu_X, sig_X)
y = ((u - mu_X) ./ sig_X);

== matlab function TFlex_SSGP/Build Common Terms/Kbf ==
  data: x1 input; K output size=[Mb,1]; x2 input; hyp input
function K = SquaredExpCov(x1,x2,hyp) %#codegen
coder.extrinsic('SEcov');
n = size(x1,1);
m = size(x2,1);
K = double(zeros(n,m));
K = SEcov(x1,x2,hyp);
end

== matlab function TFlex_SSGP/Build Common Terms/normalizeY1 ==
  data: u input; y output; mu_Y parameter; sig_Y parameter
function y = normalizeY(u,mu_Y, sig_Y)
y = ((u' - mu_Y) ./ sig_Y)';

== matlab function TFlex_SSGP/Build Common Terms/Kbf1 ==
  data: x1 input; K output; x2 input; hyp input
function K = SquaredExpCov(x1,x2,hyp) %#codegen
coder.extrinsic('SEcov');
n = size(x1,1);
m = size(x2,1);
K = double(zeros(n,m));
K = SEcov(x1,x2,hyp);
end

== matlab function TFlex_SSGP/TDfhan/MATLAB Function2 ==
  data: v1 input; output output; v2 input; r0 input; h0 input
function output = Fhan(v1,v2,r0, h0)
d = h0^2*r0;
a0 = h0*v2;
y = v1 + a0;
a1 = sqrt(d*(d+8*abs(y)));
a2 = a0 + sign(y)*(a1-d)/2;
sy = (sign(y+d)-sign(y-d))/2;
a = (a0+y-a2)*sy +a2;
sa = (sign(a+d)-sign(a-d))/2;
output = -r0 *(a/d -sign(a) )*sa - r0*sign(a);

== matlab function TFlex_SSGP/Build Common Terms/Kbf2 ==
  data: x1 input; K output; x2 input; hyp input
function K = SquaredExpCov(x1,x2,hyp) %#codegen
coder.extrinsic('SEcov');
n = size(x1,1);
m = size(x2,1);
K = double(zeros(n,m));
K = SEcov(x1,x2,hyp);
end

== matlab function TFlex_SSGP/Subsystem/normalizeX1 ==
  data: u input; y output; mu_X parameter; sig_X parameter
function y = normalizeX(u,mu_X, sig_X)
y = ((u - mu_X) ./ sig_X);

== matlab function TFlex_SSGP/Build Common Terms/Kbf3 ==
  data: x1 input; K output; x2 input; hyp input
function K = SquaredExpCov(x1,x2,hyp) %#codegen
coder.extrinsic('SEcov');
n = size(x1,1);
m = size(x2,1);
K = double(zeros(n,m));
K = SEcov(x1,x2,hyp);
end

== matlab function TFlex_SSGP/Build Common Terms/MATLAB Function1 ==
  data: K input; L output
function L = calcChol(K)
L = chol(K,'lower');

== matlab function TFlex_SSGP/Build Common Terms/Kbf4 ==
  data: x1 input; K output; x2 input; hyp input
function K = SquaredExpCov(x1,x2,hyp) %#codegen
coder.extrinsic('SEcov');
n = size(x1,1);
m = size(x2,1);
K = double(zeros(n,m));
K = SEcov(x1,x2,hyp);
end

== matlab function TFlex_SSGP/Build Common Terms/Kbf6 ==
  data: x1 input; K output; x2 input; hyp input
function K = SquaredExpCov(x1,x2,hyp) %#codegen
coder.extrinsic('SEcov');
n = size(x1,1);
m = size(x2,1);
K = double(zeros(n,m));
K = SEcov(x1,x2,hyp);
end

== matlab function TFlex_SSGP/Build Common Terms/MATLAB Function2 ==
  data: K input; L output
function L = calcChol(K)
L = chol(K,'lower');

== matlab function TFlex_SSGP/Subsystem1/MATLAB Function1 ==
  data: y input; Y data_store_memory
function writeTo(y)
global Y 

Y = [Y(2:end,:);y'];

== matlab function TFlex_SSGP/Build Common Terms/MATLAB Function4 ==
  data: K input; L output
function L = calcChol(K)
L = chol(K,'lower');

== matlab function TFlex_SSGP/Build Common Terms/normalizeX3 ==
  data: u input; y output size=[1,dof]; mu_X parameter; sig_X parameter
function y = normalizeX(u,mu_X, sig_X)
y = ((u - mu_X) ./ sig_X);

== matlab function TFlex_SSGP/Build Common Terms/Kbf5 ==
  data: x1 input; K output size=[Mb,1]; x2 input; hyp input
function K = SquaredExpCov(x1,x2,hyp) %#codegen
coder.extrinsic('SEcov');
n = size(x1,1);
m = size(x2,1);
K = double(zeros(n,m));
K = SEcov(x1,x2,hyp);
end

== matlab function TFlex_SSGP/Prediction/normalizeX3 ==
  data: u input; y output; mu_Y parameter; sig_Y parameter
function y = scaleUp(u,mu_Y, sig_Y)
y = u.*sig_Y + mu_Y;

== matlab function TFlex_SSGP/Subsystem3/MATLAB Function ==
  settings: updateMethod=DISCRETE  sampleTime=ts_opti
  data: hyp_init input; hyp_opt output; sn input; f input; yf input; a input; b input; Saa input; ma input; Kaa_old input; beta_out output; beta_init parameter; beta_min parameter; beta_reduc parameter; alpha parameter
function [hyp_opt,beta_out]= hyperparamUpdate(hyp_init,sn,f,yf,a,b,Saa,ma,Kaa_old,beta_init, beta_min, beta_reduc, alpha)
coder.extrinsic('onlineHyperUpdate_SSGP');
persistent hyp1 beta
if(isempty(hyp1))
    hyp1 = hyp_init;
    beta = beta_init;
end
hyp_opt = hyp1;
hyp_new = zeros(size(hyp_init));

hyp_new = onlineHyperUpdate_SSGP(hyp_opt,sn,alpha,f,yf,a,b,Saa,ma,Kaa_old);
hyp1 = hyp_opt.*(1-beta) + beta.*hyp_new;
hyp_opt = hyp1;


beta_new = beta.*beta_reduc;
beta = max(beta_new,beta_min);
beta_out = beta;

== matlab function TFlex_SSGP/Subsystem1/MATLAB Function2 ==
  data: x input; Y data_store_memory; X data_store_memory
function writeTo(x)
global X 

X = [X(2:end,:);x];
